simulink model "ukol3"  (R2017b)
settings: Solver=VariableStepAuto  StartTime=0.0  StopTime=10.0  RelTol=1e-3
settings Model: Creator=Milan  LastModifiedBy=ladislav
settings CodeAppCC: StateflowObjectComments=on

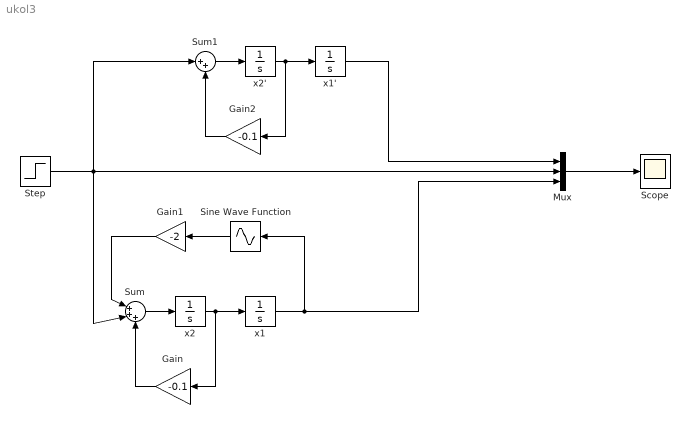
== system ukol3 ==
  Gain : Gain  Gain=-0.1
  Gain1 : Gain  Gain=-2
  Gain2 : Gain  Gain=-0.1
  Mux : Mux  Inputs=3
  "Scope " : Scope
  "Sine Wave Function " : Sin  TimeSource=Use external signal  SampleTime=0
  "Step " : Step  After=2.001  SampleTime=0
  Sum : Sum  Inputs=|+++
  Sum1 : Sum  Inputs=|++
  x1 : Integrator
  "x1' " : Integrator
  x2 : Integrator
  "x2' " : Integrator
  wires:
  "Step "/1 -> Sum1/1, Mux/2, Sum/2
  x2/1 -> Gain/1, x1/1
  Sum/1 -> x2/1
  Gain/1 -> Sum/3
  x1/1 -> Mux/3, "Sine Wave Function "/1
  "Sine Wave Function "/1 -> Gain1/1
  Gain1/1 -> Sum/1
  Mux/1 -> "Scope "/1
  Sum1/1 -> "x2' "/1
  "x2' "/1 -> Gain2/1, "x1' "/1
  Gain2/1 -> Sum1/2
  "x1' "/1 -> Mux/1
